simulink model "lab3_2"  (R2017a)
settings: Solver=VariableStepAuto  StartTime=0.0  StopTime=20  RelTol=1e-3
libraries: commchan3 x1
settings Model: Creator=Mikle  LastModifiedBy=Mikle

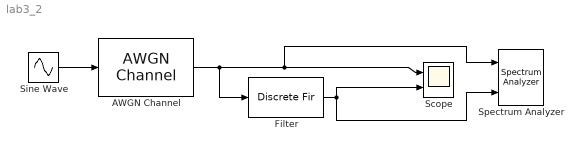
== system lab3_2 ==
  AWGN Channel : commchan3/AWGN Channel  InputProcessing=Columns as channels (frame based)  seed=67  noiseMode="Signal to noise ratio  (Eb/No)"  EbNodB=10  EsNodB=10  SNRdB=10  bitsPerSym=1  Ps=1  Tsym=1  variance=1
  Filter : DiscreteFir  Tag=BlockMethodSubSystem  Coefficients=[-0.0019228147313446857 -0.0019196158753200987 -0.0019144168146620598 -0.0019071899628651237 -0.0018979089640780533 -0.0018865487228950878 -0.0018730854333011344 -0.0018574966067423484 -0.0018397610992942019 -0.0018198591378998175 -0.0017977723456520486 -0.0017734837660934937 -0.0017469778865093753 -0.0017182406601890371 -0.001687259527632539 -0.0016540234366797144 -0.0016185228615398573 -0.001580749820701093 -0.0015406978936993812 -0.0014983622367279853 -0.0014537395970691924 -0.0014068283263310173 -0.0013576283924725692 -0.0013061413906027798 -0.0012523705525381503 -0.0011963207551062413 -0.0011379985271826106 -0.0010774120554499919 -0.0010145711888695568 -0.00094948744185514606 -0.00088217399614248142 -0.00081264570134644779 -0.00074091907420061173 -0.00066701229647430943 -0.00059094521156368926 -0.00051273931975429326 -0.00043241777215380974 -0.00035000536329485592 -0.00026552852240869433 -0.00017901530337201754 -9.0495373329995654e-05 3.5657464592718348e-19 9.2437962338516569e-05 0.00018678408816128817 0.00028300239731588009 0.00038105537292878203 0.00048090398059286632 0.00058250768882406681 0.00068582449077495065 0.00079081092719179814 0.00089742211060067374 0.0010056117507069215 0.0011153321809913728 0.0012265343864855836 0.001339168032707262 0.0014531814957361091 0.0015685218934091676 0.0016851351176138836 0.0018029658676559633 0.0019219576846782726 0.0020420529871059299 0.0021631931070919489 0.0022853183279367465 0.0024083679224540413 0.0025322801922547139 0.0026569925079194209 0.0027824413500298711 0.002908562351027938 0.0030352903378709209 0.0031625593754506121 0.0032903028107430518 0.0034184533176551566 0.0035469429425337706 0.0036757031503020349 0.0038046648711873477 0.0039337585480046511 0.004062914183958221 0.0041920613909245397 0.0043211294381785247 0.0044500473015247344 0.0045787437127949131 0.0047071472096727367 0.0048351861858063521 0.0049627889411689372 0.0050898837326272236 0.0052163988246777121 0.0053422625403100653 0.0054674033119569421 0.0055917497324895126 0.0057152306062176446 0.0058377749998537896 0.0059593122933994502 0.0060797722309132319 0.0061990849711194024 0.0063171811378160206 0.0064339918700417774 0.0065494488719607929 0.0066634844624249168 0.0067760316241730727 0.0068870240526277098 0.0069963962042484127 0.0071040833444032982 0.0072100215947189829 0.0073141479798704313 0.0074164004737723053 0.0075167180451339594 0.007615040702340683 0.0077113095376243343 0.0078054667704870184 0.0078974557903421019 0.0079872211983373874 0.0080747088483260811 0.0081598658869516394 0.0082426407928134632 0.0083229834146811114 0.0084008450087253717 0.0084761782747354748 0.0085489373912924164 0.0086190780498692967 0.0086865574878304038 0.008751334520301678 0.0088133695708861644 0.0088726247011989227 0.0089290636391968613 0.0089826518062800422 0.0090333563431418545 0.0090811461343465929 0.0091259918316140658 0.0091678658757917454 0.0092067425174963014 0.0092425978364072403 0.0092754097591966518 0.0093051580760800945 0.0093318244559748523 0.0093553924602529179 0.0093758475550772564 0.0093931771223110545 0.0094073704689908826 0.0094184188353558292 0.0094263154014259734 0.0094310552921246463 0.0094326355809402646 0.0094310552921246463 0.0094263154014259734 0.0094184188353558292 0.0094073704689908826 0.0093931771223110545 0.0093758475550772564 0.0093553924602529179 0.0093318244559748523 0.0093051580760800945 0.0092754097591966518 0.0092425978364072403 0.0092067425174963014 0.0091678658757917454 0.0091259918316140658 0.0090811461343465929 0.0090333563431418545 0.0089826518062800422 0.0089290636391968613 0.0088726247011989227 0.0088133695708861644 0.008751334520301678 0.0086865574878304038 0.0086190780498692967 0.0085489373912924164 0.0084761782747354748 0.0084008450087253717 0.0083229834146811114 0.0082426407928134632 0.0081598658869516394 0.0080747088483260811 0.0079872211983373874 0.0078974557903421019 0.0078054667704870184 0.0077113095376243343 0.007615040702340683 0.0075167180451339594 0.0074164004737723053 ...(+2346 chars)]  InputProcessing=Columns as channels (frame based)
  Scope : Scope  NumInputPorts=2
  Sine Wave : Sin  SampleTime=0.01
  Spectrum Analyzer : SpectrumAnalyzer  NumInputPorts=2
  wires:
  AWGN Channel/1 -> Filter/1, Spectrum Analyzer/1, Scope/1
  Sine Wave/1 -> AWGN Channel/1
  Filter/1 -> Spectrum Analyzer/2, Scope/2
